simulink model "slidingmodecontrol"  (R2021a)
settings: Solver=ode4  StartTime=0.0  StopTime=100  FixedStep=0.02  RelTol=1e-3
values from neighbouring files (symbols this model uses):
  deltar = 0.005    [Ini_SO3.m]    (also in Ini_SO3_MixedCZ.m = 0.01; Ini_Usat.m = 0.01)
  deltat = 0.02    [Ini_SO3_MixedCZ.m]    (also in Ini_Usat.m)
  R = 1    [Ini_SO3.m]    (also in Ini_SO3_MixedCZ.m = 2; Ini_Usat.m = 2; SO3.m = eye(3)+(1-cos(ang))*x2x_hat(x)*x2x_hat(x)+sin(ang)*x2x_hat(x; plot2D.m = tran(lamda_con(j),phi_con(j)))
undefined symbols (not defined in the file or in its folder): deg, rad, s
libraries: aerolibconvert2 x1
settings Model: Creator=Zeyu  LastModifiedBy=泽禹
settings SolverCC: AlgebraicLoopSolver=TrustRegion
settings OptimizationCC: LifeSpan=inf
settings DebuggingCC: SFMachineParentedDataDiag=warning  UnderSpecifiedDimensionMsg=warning  ArithmeticOperatorsInVariantConditions=warning
settings SFSimCC: CustomCodeUndefinedFunction=UseInterfaceOnly
settings CodeAppCC: StateflowObjectComments=on

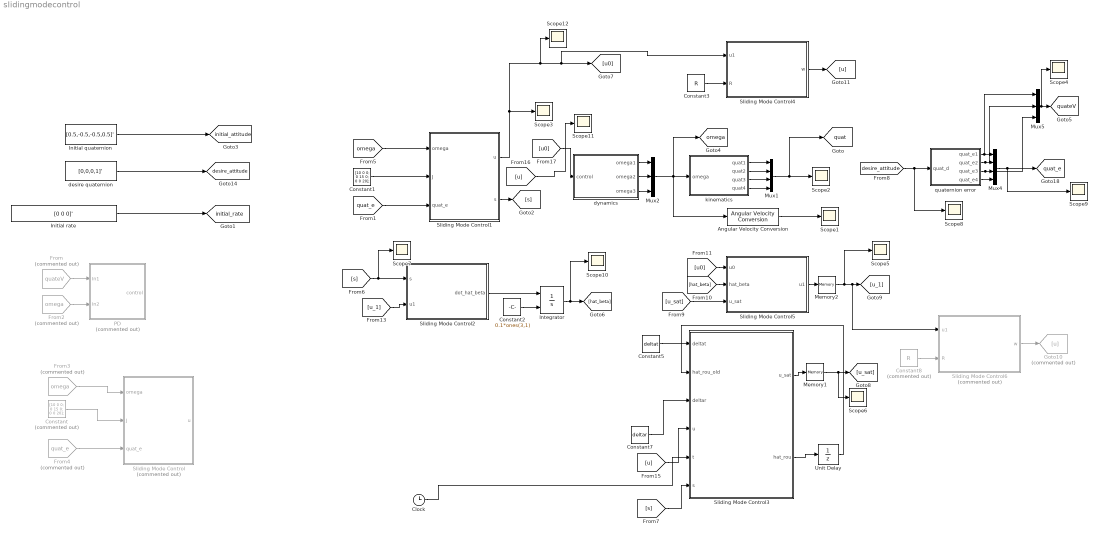
== system slidingmodecontrol ==
  Angular Velocity Conversion : aerolibconvert2/Angular Velocity Conversion  IU=rad/s  OU=deg/s
  Clock : Clock
  Constant : Constant  Commented=on  Value=|
      | [10 0 0;
      |     0 15 0;
      |     0 0 20];
  Constant1 : Constant  Value=|
      | [10 0 0;
      |     0 15 0;
      |     0 0 20];
  Constant2 : Constant  Value=0.1*ones(3,1)
  Constant3 : Constant  Value=R
  Constant5 : Constant  Value=deltat
  Constant7 : Constant  Value=deltar
  Constant8 : Constant  Commented=on  Value=R
  From : From  Commented=on  GotoTag=quateV  TagVisibility=global
  From2 : From  Commented=on  GotoTag=omega  TagVisibility=global
  From3 : From  Commented=on  GotoTag=omega  TagVisibility=global
  From4 : From  Commented=on  GotoTag=quat_e  TagVisibility=global
  Goto10 : Goto  Commented=on  GotoTag=u
  Initial quaternion : Constant  Value=[0.5,-0.5,-0.5,0.5]'
  Initial rate : Constant  Value=[0 0 0]'  VectorParams1D=off
  Integrator : Integrator  InitialConditionSource=external
  Memory1 : Memory
  Memory2 : Memory
  Mux1 : Mux
  Mux2 : Mux  Inputs=3
  Mux4 : Mux
  Mux5 : Mux  Inputs=3
  PD : Subsystem  Commented=on
  Scope{1..12} (12 alike) : Scope
  Sliding Mode Control : MATLAB Function  Commented=on  TreatAsAtomicUnit=on
  Sliding Mode Control1 : MATLAB Function  TreatAsAtomicUnit=on
  Sliding Mode Control2 : MATLAB Function  TreatAsAtomicUnit=on
  Sliding Mode Control3 : MATLAB Function  TreatAsAtomicUnit=on
  Sliding Mode Control4 : MATLAB Function  TreatAsAtomicUnit=on
  Sliding Mode Control5 : MATLAB Function  TreatAsAtomicUnit=on
  Sliding Mode Control6 : MATLAB Function  Commented=on  TreatAsAtomicUnit=on
  Unit Delay : UnitDelay  InitialCondition=zeros(3,R/deltar)  SampleTime=-1  HasFrameUpgradeWarning=on
  desire quaternion : Constant  Value=[0,0,0,1]'
  dynamics : Subsystem
  kinematics : Subsystem
  quaternion error : Subsystem
  tag scope: desire_attitude=global, initial_attitude=global, initial_rate=global, omega=global, quat=global, quat_e=global, quateV=global
  wires:
  quaternion error/4(quat_e4) -> Mux4/4
  dynamics/3(omega3) -> Mux2/3
  Mux1/1 -> Scope2/1, [quat]
  Mux4/1 -> Scope9/1, [quat_e]
  kinematics/3(quat3) -> Mux1/3
  dynamics/1(omega1) -> Mux2/1
  kinematics/1(quat1) -> Mux1/1
  Mux2/1 -> Angular Velocity Conversion/1, [omega], kinematics/1(omega)
  kinematics/4(quat4) -> Mux1/4
  Angular Velocity Conversion/1 -> Scope1/1
  dynamics/2(omega2) -> Mux2/2
  [desire_attitude] -> Scope8/1, quaternion error/1(quat_d)
  kinematics/2(quat2) -> Mux1/2
  Initial quaternion/1 -> [initial_attitude]
  desire quaternion/1 -> [desire_attitude]
  Initial rate/1 -> [initial_rate]
  From/1 -> PD/1(In1)
  From2/1 -> PD/2(In2)
  Mux5/1 -> Scope4/1, [quateV]
  quaternion error/2(quat_e2) -> Mux5/2, Mux4/2
  quaternion error/1(quat_e1) -> Mux5/1, Mux4/1
  quaternion error/3(quat_e3) -> Mux5/3, Mux4/3
  From3/1 -> Sliding Mode Control/1(omega)
  From4/1 -> Sliding Mode Control/3(quat_e)
  Constant/1 -> Sliding Mode Control/2(J)
  [quat_e] -> Sliding Mode Control1/3(quat_e)
  Constant1/1 -> Sliding Mode Control1/2(J)
  [omega] -> Sliding Mode Control1/1(omega)
  Sliding Mode Control1/2(s) -> [s]
  [s] -> Scope7/1, Sliding Mode Control2/1(s)
  Sliding Mode Control2/1(dot_hat_beta) -> Integrator/1
  Constant2/1 -> Integrator/2
  Integrator/1 -> Scope10/1, [hat_beta]
  Sliding Mode Control3/2(hat_rou) -> Unit Delay/1
  Sliding Mode Control3/1(u_sat) -> Memory1/1
  [hat_beta] -> Sliding Mode Control5/2(hat_beta)
  [u0] -> Sliding Mode Control5/1(u0)
  Sliding Mode Control5/1(u1) -> Memory2/1
  [u_1] -> Sliding Mode Control2/2(u1)
  Constant5/1 -> Sliding Mode Control3/1(deltat)
  Constant7/1 -> Sliding Mode Control3/3(deltar)
  Clock/1 -> Sliding Mode Control3/5(t)
  [u_sat] -> Sliding Mode Control5/3(u_sat)
  Unit Delay/1 -> Sliding Mode Control3/2(hat_rou_old)
  [u] -> Sliding Mode Control3/4(u)
  Memory1/1 -> Scope6/1, [u_sat]
  Memory2/1 -> Scope5/1, Sliding Mode Control6/1(u1), [u_1]
  Constant8/1 -> Sliding Mode Control6/2(R)
  Sliding Mode Control6/1(w) -> Goto10/1
  Sliding Mode Control1/1(u) -> Sliding Mode Control4/1(u1), [u0], Scope12/1, Scope3/1
  [u] -> Scope11/1
  [s] -> Sliding Mode Control3/6(s)
  Constant3/1 -> Sliding Mode Control4/2(R)
  Sliding Mode Control4/1(w) -> [u]
  [u0] -> dynamics/1(control)

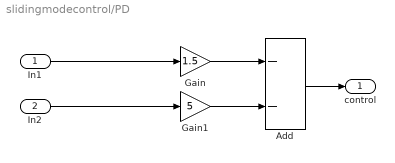
== system slidingmodecontrol/PD ==
  In1 : Inport
  In2 : Inport  Port=2
  Add : Sum  Inputs=--
  Gain : Gain  Gain=1.5
  Gain1 : Gain  Gain=5
  control : Outport
  wires:
  Gain/1 -> Add/1
  In1/1 -> Gain/1
  In2/1 -> Gain1/1
  Gain1/1 -> Add/2
  Add/1 -> control/1

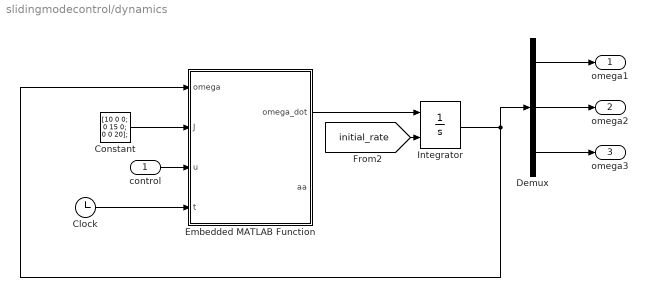
== system slidingmodecontrol/dynamics ==
  control : Inport
  Clock : Clock
  Constant : Constant  Value=|
      | [10 0 0;
      |     0 15 0;
      |     0 0 20];
  Demux : Demux  Outputs=3
  Embedded MATLAB Function : MATLAB Function  TreatAsAtomicUnit=on
  Integrator : Integrator  InitialConditionSource=external
  omega1 : Outport
  omega2 : Outport  Port=2
  omega3 : Outport  Port=3
  wires:
  Embedded MATLAB Function/1(omega_dot) -> Integrator/1
  Integrator/1 -> Demux/1, Embedded MATLAB Function/1(omega)
  Demux/1 -> omega1/1
  Demux/2 -> omega2/1
  Demux/3 -> omega3/1
  Constant/1 -> Embedded MATLAB Function/2(J)
  control/1 -> Embedded MATLAB Function/3(u)
  Clock/1 -> Embedded MATLAB Function/4(t)
  [initial_rate] -> Integrator/2

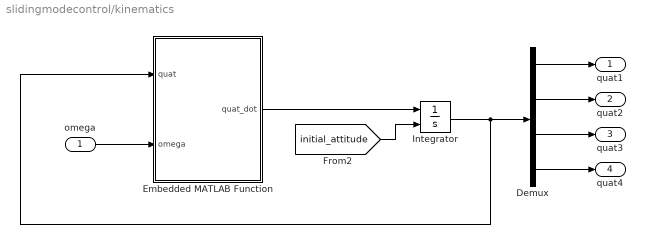
== system slidingmodecontrol/kinematics ==
  omega : Inport
  Demux : Demux
  Embedded MATLAB Function : MATLAB Function  TreatAsAtomicUnit=on
  Integrator : Integrator  InitialConditionSource=external
  quat1 : Outport
  quat2 : Outport  Port=2
  quat3 : Outport  Port=3
  quat4 : Outport  Port=4
  wires:
  Embedded MATLAB Function/1(quat_dot) -> Integrator/1
  Integrator/1 -> Embedded MATLAB Function/1(quat), Demux/1
  Demux/1 -> quat1/1
  Demux/2 -> quat2/1
  Demux/3 -> quat3/1
  omega/1 -> Embedded MATLAB Function/2(omega)
  Demux/4 -> quat4/1
  [initial_attitude] -> Integrator/2

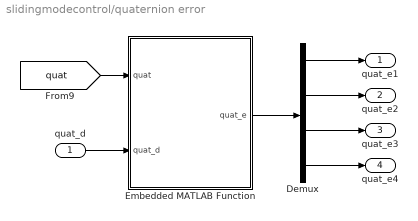
== system slidingmodecontrol/quaternion error ==
  quat_d : Inport
  Demux : Demux
  Embedded MATLAB Function : MATLAB Function  TreatAsAtomicUnit=on
  quat_e1 : Outport
  quat_e2 : Outport  Port=2
  quat_e3 : Outport  Port=3
  quat_e4 : Outport  Port=4
  wires:
  quat_d/1 -> Embedded MATLAB Function/2(quat_d)
  [quat] -> Embedded MATLAB Function/1(quat)
  Embedded MATLAB Function/1(quat_e) -> Demux/1
  Demux/1 -> quat_e1/1
  Demux/2 -> quat_e2/1
  Demux/3 -> quat_e3/1
  Demux/4 -> quat_e4/1

== matlab function slidingmodecontrol/Sliding Mode Control6 ==
  data: u1 input; w output; R input
function w  = fcn(u1,R)
    w=zeros(3,1);
    if u1(1)>=R
        w(1)=1;
    end
    if u1(1)>0 && u1(1)<R
        w(1)=u1(1)-1/4*u1(1)^2;
    end
    if u1(1)>R
        w(1)=1;
    end
    if u1(1)<=-R
        w(1)=-1;
    end
    if u1(1)<0 && u1(1)>-R
        w(1)=u1(1)+1/4*u1(1)^2;
    end
    %% 
    if u1(2)>=R
        w(2)=1;
    end
    if u1(2)>0 && u1(2)<R
        w(2)=u1(2)-1/4*u1(2)^2;
    end
    if u1(2)>R
        w(2)=1;
    end
    if u1(2)<=-R
        w(2)=-1;
    end
    if u1(2)<0 && u1(2)>-R
        w(2)=u1(2)+1/4*u1(2)^2;
    end
    
    %% 
    if u1(3)>=R
        w(3)=1;
    end
    if u1(3)>0 && u1(3)<R
        w(3)=u1(3)-1/4*u1(3)^2;
    end
    if u1(3)>R
        w(3)=1;
    end
    if u1(3)<=-R
        w(3)=-1;
    end
    if u1(3)<0 && u1(3)>-R
        w(3)=u1(3)+1/4*u1(3)^2;
    end
end

== matlab function slidingmodecontrol/quaternion error/Embedded MATLAB Function ==
  data: quat input; quat_d input; quat_e output
function quat_e = fcn(quat,quat_d)
% This block supports the Embedded MATLAB subset.
% See the help menu for details. 

quat_d_inv = [ -quat_d(1), -quat_d(2), -quat_d(3), quat_d(4)]';

quat_e = Quat_Prodct(quat_d_inv,quat);

== matlab function slidingmodecontrol/Sliding Mode Control ==
  data: omega input; u output; J input; quat_e input
function u  = fcn(omega, J, quat_e)

c=1;L=0.06;alpha=0.1;

omega_x = [0            -omega(3)       omega(2);
           omega(3)     0               -omega(1);
           -omega(2)    omega(1)        0       ]; 
quat_e_x = [0            -quat_e(3)       quat_e(2);
           quat_e(3)     0               -quat_e(1);
           -quat_e(2)    quat_e(1)        0       ]; 
s=omega+c*quat_e(1:3);
u=omega_x*J*omega-J*(c/2*(quat_e_x+quat_e(4)*eye(3))*omega)-(L*norm(inv(J))+alpha/sqrt(2))*J*sign(s);

== matlab function slidingmodecontrol/dynamics/Embedded MATLAB Function ==
  data: omega input; omega_dot output; J input; u input; t input; aa output
function [omega_dot,aa]  = fcn(omega, J, u, t)
% This block supports the Embedded MATLAB subset.
% See the help menu for details. 


omega_x = [0            -omega(3)       omega(2);
           omega(3)     0               -omega(1);
           -omega(2)    omega(1)        0       ]; 


% d = [ 0.05*sin(pi/10*t);
%       0.03*sin(pi/20*t);
%       0.06*sin(pi/20*t)];

omega_dot = inv(J) * ( -omega_x*J*omega + u);
aa=-omega_x*J*omega + u;

== matlab function slidingmodecontrol/Sliding Mode Control1 ==
  data: omega input; u output; J input; quat_e input; s output
function [u,s]  = fcn(omega, J, quat_e)

k=2;k1=2;ksi=0.01;
% k=3;k1=3;ksi=0.01;  直接加饱和 限制久，但通过自适应方法 比较柔和 稳定

omega_x = [0            -omega(3)       omega(2);
           omega(3)     0               -omega(1);
           -omega(2)    omega(1)        0       ]; 
quat_e_x = [0            -quat_e(3)       quat_e(2);
           quat_e(3)     0               -quat_e(1);
           -quat_e(2)    quat_e(1)        0       ]; 
s=omega+k*quat_e(1:3);
u=omega_x*J*omega-k1*s+2*k*k1*quat_e(1:3)'*omega*(s/(norm(s)+0.01)^2)-J*(k/2*(quat_e_x+quat_e(4)*eye(3))*omega);
% u=omega_x*J*omega-J*(c/2*(quat_e_x+quat_e(4)*eye(3))*omega)-(L*norm(inv(J))+alpha/sqrt(2))*J*(s/(norm(s)+0.01));

== matlab function slidingmodecontrol/Sliding Mode Control2 ==
  data: s input; dot_hat_beta output; u1 input
function dot_hat_beta  = fcn(s,u1)
dot_hat_beta=zeros(3,1);
k_beta=0.05;

dot_hat_beta(1) = -k_beta*s(1)*u1(1);
dot_hat_beta(2) = -k_beta*s(2)*u1(2);
dot_hat_beta(3) = -k_beta*s(3)*u1(3);

== matlab function slidingmodecontrol/Sliding Mode Control3 ==
  data: deltat input; u_sat output; hat_rou_old input; deltar input; hat_rou output; u input; t input; s input
function [u_sat,hat_rou]  = fcn(deltat,hat_rou_old,deltar,u,t,s)
     N=200;
     hat_rou=zeros(3,N);
     u_sat_temp=zeros(3,N);
     u_sat=zeros(3,1);
     
     k_rou=0.005;
     dot_hat_rou =zeros(3,N);
     if t==0
        dot_hat_rou =zeros(3,N);
     else
        for i=1:N
        dot_hat_rou(1,i)=k_rou*s(1)*DeadZone(i*deltar,u(1));
        dot_hat_rou(2,i)=k_rou*s(2)*DeadZone(i*deltar,u(2));
        dot_hat_rou(3,i)=k_rou*s(3)*DeadZone(i*deltar,u(3));
        end
     end
     
     if t==0
        hat_rou=zeros(3,N); 
        u_sat=zeros(3,1);
     else
        for i=1:N
         hat_rou(1,i)=deltat*dot_hat_rou(1,i)+hat_rou_old(1,i);
         hat_rou(2,i)=deltat*dot_hat_rou(2,i)+hat_rou_old(2,i);
         hat_rou(3,i)=deltat*dot_hat_rou(3,i)+hat_rou_old(3,i);
%          u_sat_temp(1,i)= hat_rou(1,i)*DeadZone(i*deltar,u(1));
%          u_sat_temp(2,i)= hat_rou(2,i)*DeadZone(i*deltar,u(2));
%          u_sat_temp(3,i)= hat_rou(3,i)*DeadZone(i*deltar,u(3));
         u_sat_temp(1,i)= hat_rou(1,i);
         u_sat_temp(2,i)= hat_rou(2,i);
         u_sat_temp(3,i)= hat_rou(3,i);
        end
        u_sat(1)=sum(u_sat_temp(1,:))*deltar;
        u_sat(2)=sum(u_sat_temp(2,:))*deltar;
        u_sat(3)=sum(u_sat_temp(3,:))*deltar; 
     end
     
     
end

== matlab function slidingmodecontrol/Sliding Mode Control4 ==
  data: u1 input; w output; R input
function w  = fcn(u1,R)
    w=zeros(3,1);
    if u1(1)>=R
        w(1)=1;
    end
    if u1(1)>0 && u1(1)<R
        w(1)=u1(1)-1/4*u1(1)^2;
    end
    if u1(1)>R
        w(1)=1;
    end
    if u1(1)<=-R
        w(1)=-1;
    end
    if u1(1)<0 && u1(1)>-R
        w(1)=u1(1)+1/4*u1(1)^2;
    end
    %% 
    if u1(2)>=R
        w(2)=1;
    end
    if u1(2)>0 && u1(2)<R
        w(2)=u1(2)-1/4*u1(2)^2;
    end
    if u1(2)>R
        w(2)=1;
    end
    if u1(2)<=-R
        w(2)=-1;
    end
    if u1(2)<0 && u1(2)>-R
        w(2)=u1(2)+1/4*u1(2)^2;
    end
    
    %% 
    if u1(3)>=R
        w(3)=1;
    end
    if u1(3)>0 && u1(3)<R
        w(3)=u1(3)-1/4*u1(3)^2;
    end
    if u1(3)>R
        w(3)=1;
    end
    if u1(3)<=-R
        w(3)=-1;
    end
    if u1(3)<0 && u1(3)>-R
        w(3)=u1(3)+1/4*u1(3)^2;
    end
end

== matlab function slidingmodecontrol/Sliding Mode Control5 ==
  data: u0 input; u1 output; hat_beta input; u_sat input
function u1  = fcn(u0,hat_beta,u_sat)
 u1=zeros(3,1);
 u1_temp=u0-u_sat;
u1(1)=hat_beta(1)*u1_temp(1);
u1(2)=hat_beta(2)*u1_temp(2);
u1(3)=hat_beta(3)*u1_temp(3);

== matlab function slidingmodecontrol/kinematics/Embedded MATLAB Function ==
  data: quat input; omega input; quat_dot output
function quat_dot = fcn(quat,omega)
% This block supports the Embedded MATLAB subset.
% See the help menu for details. 
quat13 = quat(1:3);
quat13_x = [0             -quat(3)        quat(2);
            quat(3)       0               -quat(1);
            -quat(2)      quat(1)         0];

F13 = 0.5*(quat13_x+quat(4)*eye(3));
F4 = -0.5*quat13';
F = [F13;F4];

quat_dot = F*omega ;
